simulink model "first_version"  (R2021b)
settings: Solver=FixedStepDiscrete  StartTime=0.0  StopTime=10.0  FixedStep=0.1  RelTol=1e-3  EnableMultiTasking=on
undefined symbols (not defined in the file): m, n
settings Model: Creator=mattiabacci  LastModifiedBy=mattiabacci
settings SolverCC: AlgebraicLoopSolver=TrustRegion  AutoInsertRateTranBlk=on
settings DataIOCC: LimitDataPoints=on
settings OptimizationCC: LifeSpan=inf
settings DebuggingCC: AllowSymbolicDim=off  SFUnexpectedBacktrackingDiag=warning  SFNoUnconditionalDefaultTransitionDiag=warning  SFExecutionAtInitializationDiag=none  ArithmeticOperatorsInVariantConditions=warning
settings SFSimCC: SimUseLocalCustomCode=off  CustomCodeUndefinedFunction=UseInterfaceOnly
settings RTWCC: RTWUseLocalCustomCode=off
settings CodeAppCC: StateflowObjectComments=on
settings GRTTargetCC: TargetLangStandard=C89/C90 (ANSI)
settings ConfigComp: CovMetricSettings=dw  CovSaveCumulativeToWorkspaceVar=on  CovSaveSingleToWorkspaceVar=on  CovExternalEMLEnable=off  CovSFcnEnable=off

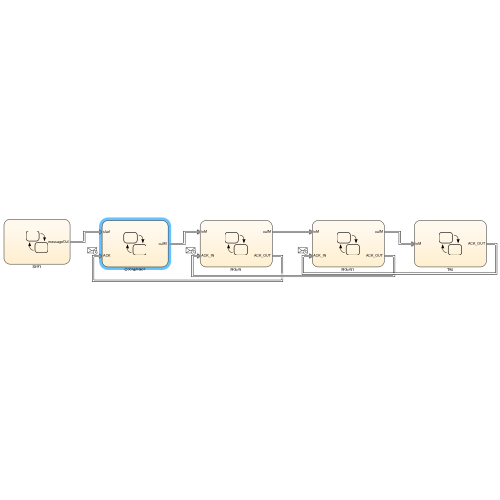
[thumbnail: Simulink's stored preview of the top-level diagram]
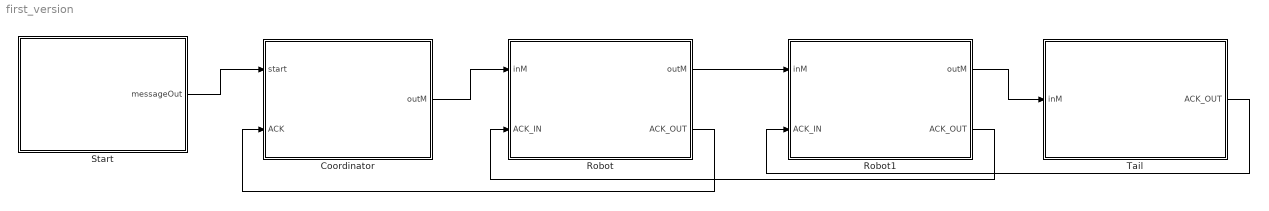
== system first_version ==
  Coordinator : Stateflow chart  TreatAsAtomicUnit=on
  Robot : Stateflow chart  TreatAsAtomicUnit=on
  Robot1 : Stateflow chart  TreatAsAtomicUnit=on
  Start : Stateflow chart  TreatAsAtomicUnit=on
  Tail : Stateflow chart  TreatAsAtomicUnit=on
  wires:
  Start/1(messageOut) -> Coordinator/1(start)
  Coordinator/1(outM) -> Robot/1(inM)
  Robot/2(ACK_OUT) -> Coordinator/2(ACK)
  Robot/1(outM) -> Robot1/1(inM)
  Robot1/2(ACK_OUT) -> Robot/2(ACK_IN)
  Robot1/1(outM) -> Tail/1(inM)
  Tail/1(ACK_OUT) -> Robot1/2(ACK_IN)

== stateflow chart first_version/Start ==
  state Begin
    entry:
    messageOut.data = 1;
    send(messageOut);
  (default) -> Begin
  data: messageOut output

== stateflow chart first_version/Robot1 ==
  state Decision
    entry:
    m_now= inM.data(1);
    m_target= inM.data(2);
    n= inM.data(3);
    randN = Random();
    if randN > 0.5
    m_now = m_now + 1;
    end
  state Begin
    entry:
    flag=0
  state ACK
    entry:
    ACK_OUT.data = ACK_IN.data;
    send(ACK_OUT);
  state OutputInterface
    entry:
    if m_now==m_target
    ACK_OUT.data = 1;
    send(ACK_OUT);
    else
    out=[0,m_target, n];
    out(1) = m_now;
    outM.data=out;
    send(outM);
    end
  (default) -> Begin
  Begin -> Decision [order 1] : inM
  OutputInterface -> Begin
  ACK -> Begin
  Begin -> ACK [order 2] : ACK_IN
  Decision -> OutputInterface
  data: r function_output; m_now local; m_target local; n local; out local; randN local; outM output size=[1 3]; flag local; inM input size=3; ACK_IN input; ACK_OUT output
  function r = Random:
    | function r = Random
    | %#codegen
    | r = rand(1);
    | end

== stateflow chart first_version/Tail ==
  state Decision
    entry:
    m_now= inM.data(1);
    m_target= inM.data(2);
    n= inM.data(3);
    randN = Random();
    if randN > 0.5
    m_now = m_now + 1;
    end
  state Begin
    entry:
    flag=0
  state OutputInterface
    entry:
    if m_now==m_target
    ACK_OUT.data = 1;
    send(ACK_OUT);
    else
    ACK_OUT.data = -1;
    send(ACK_OUT);
    end
  (default) -> Begin
  Begin -> Decision : inM
  OutputInterface -> Begin
  Decision -> OutputInterface
  data: r function_output; m_now local; m_target local; n local; randN local; flag local; inM input size=3; ACK_OUT output
  function r = Random:
    | function r = Random
    | %#codegen
    | r = rand(1);
    | end

== stateflow chart first_version/Robot ==
  state Begin
    entry:
    flag=0
  state Decision
    entry:
    m_now= inM.data(1);
    m_target= inM.data(2);
    n= inM.data(3);
    randN = Random();
    if randN > 0.5
    m_now = m_now + 1;
    end
  state ACK
    entry:
    ACK_OUT.data = ACK_IN.data;
    send(ACK_OUT);
  state OutputInterface
    entry:
    if m_now==m_target
    ACK_OUT.data = 1;
    send(ACK_OUT);
    else
    out=[0,m_target, n];
    out(1) = m_now;
    outM.data=out;
    send(outM);
    end
  (default) -> Begin
  Begin -> Decision [order 1] : inM
  OutputInterface -> Begin
  ACK -> Begin
  Begin -> ACK [order 2] : ACK_IN
  Decision -> OutputInterface
  data: r function_output; m_now local; m_target local; n local; out local; randN local; outM output size=[1 3]; flag local; inM input size=3; ACK_IN input; ACK_OUT output
  function r = Random:
    | function r = Random
    | %#codegen
    | r = rand(1);
    | end

== stateflow chart first_version/Coordinator ==
  state Begin
    entry:
  state Decision
    entry:
    randN = Random();
    out=[0,m_target, n];
    if randN > 0.5
    m_now = m_now + 1;
    end
    out(1) = m_now;
    outM.data=out;
    send(outM);
  state ACK
    entry:
    ackValue= ACK.data;
  (default) -> Begin : {m_now=0,
      | m_target=3,
      | n=4}
  Begin -> Decision [order 1] : start
  Decision -> Begin
  ACK -> Begin
  Begin -> ACK [order 2] : ACK
  data: r function_output; start input; randN local; m_now local; n local; m_target local; flag local; out local; outM output size=[1 3]; ACK input; ackValue local
  function r = Random:
    | function r = Random
    | %#codegen
    | r = rand(1);
    | end
